simulink model "combined_models_v16"  (R2021a)
settings: Solver=VariableStepAuto  StartTime=0.0  StopTime=30  RelTol=1e-3
values from neighbouring files (symbols this model uses):
  r__s_st = r__s_stCG - r__t_tCG    [init_saildrone_dynamics_v5.m]    (also in moduleBasedModel_v7.m = cfg.r__s_st; systemVelocities.m = cfg.r__s_st)
  r__t_tAC = r__t_tCG    [init_saildrone_dynamics_v5.m]
  rho = 1025    [init_saildrone_dynamics_v5.m]    (also in moduleBasedModel_v7.m = cfg.rho; simplifiedModel_v8.m = cfg.rho)
  rho_air = 1.225    [init_saildrone_dynamics_v5.m]
undefined symbols (not defined in the file or in its folder): beta_V_w, cfg, delta_LOS, DiscIntNeverNeededParam, gamma_c, GWP, heading_controller_samplingtime, heading_rate_ref, K_b, K_d_heading, K_d_heading2, K_d_s, k_d_s, K_d_t, K_i_heading, K_i_heading2, K_i_s, k_i_s, K_i_t, K_p_heading, K_p_heading2, k_p_s, K_p_s, K_p_t, Ka_lin, keel, ObjectsPosition, omega_n_heading2, omega_n_s, q0, q_dot0, rudder, sail, sail_AOA_controller_samplingtime, sail_AOA_linearization_point, sail_AOA_saturation, sail_AOA_table, simulation_sampling_time, start_w_trans, tacking_minus, tacking_plus, tail, theta0, timeconstant_w, U_c, U_linearization_heading, U_w, U_w_step, v_current, v_wind, v_wind_unit, wn_ref_heading, wn_ref_t, xi0, zeta_ref_heading, zeta_ref_t
(part 2 of 3)

== system combined_models_v16/Subsystem/1st order rudder dynamics ==
  note: Create smooth saturation limits
  note: Positive rudder command
      | give positive heading angle
  note: Saturate angle input, so the derivative converge to 0 at saturation,
      | LP filter in order to maintain reasonable angular velocities
  delta_r0 : Inport
  delta_r_d : Inport  Port=2
  1/time constant : Gain  Gain=1/cfg.rudder_time_constant
  Integrator5 : Integrator  InitialConditionSource=external  InitialCondition=0.5
  Pos rudder give pos yaw : Gain  Gain=-1
  Saturation : Saturate  UpperLimit=cfg.rudder_saturation_limit  LowerLimit=-cfg.rudder_saturation_limit
  Saturation1 : Saturate  UpperLimit=cfg.rudder_saturation_limit  LowerLimit=-cfg.rudder_saturation_limit
  Sum6 : Sum  Inputs=|+-
  Transfer Fcn : TransferFcn  Denominator=[cfg.rudder_time_constant/10 1]
  Transfer Fcn1 : TransferFcn  Denominator=[cfg.rudder_time_constant/10 1]
  rudder gain : Gain  Gain=cfg.rudder_gain
  delta_r_dot : Outport
  delta_r : Outport  Port=2
  wires:
  Sum6/1 -> 1/time constant/1
  Integrator5/1 -> Saturation/1
  delta_r0/1 -> Integrator5/2
  delta_r_d/1 -> Pos rudder give pos yaw/1
  Saturation/1 -> Transfer Fcn/1
  Transfer Fcn/1 -> Sum6/2, delta_r/1
  Pos rudder give pos yaw/1 -> rudder gain/1
  1/time constant/1 -> delta_r_dot/1, Integrator5/1  "delta_r_dot"
  rudder gain/1 -> Saturation1/1
  Saturation1/1 -> Transfer Fcn1/1
  Transfer Fcn1/1 -> Sum6/1

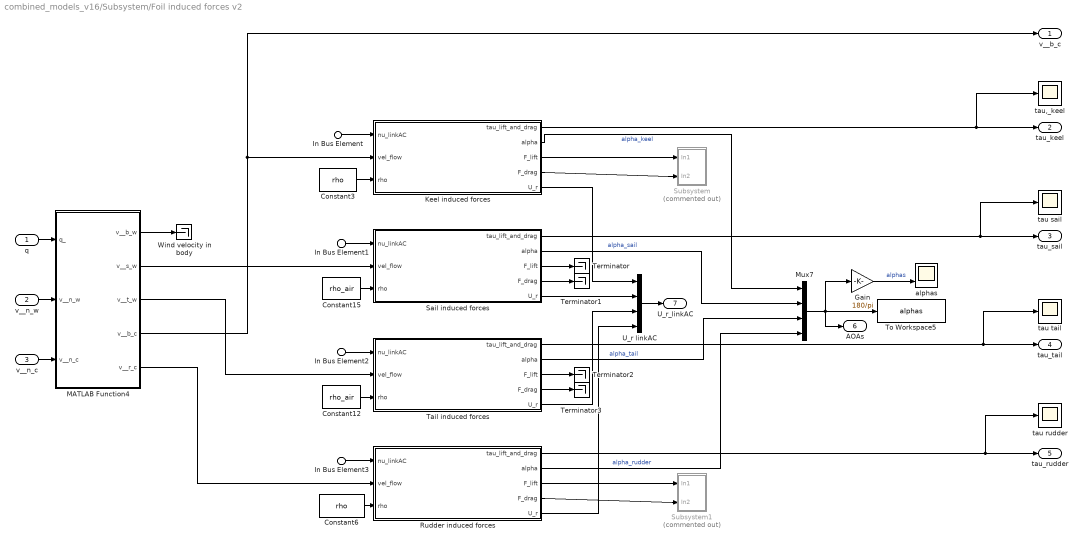
== system combined_models_v16/Subsystem/Foil induced forces v2 ==
  q : Inport
  v__n_w : Inport  Port=2
  v__n_c : Inport  Port=3
  In Bus Element : Inport  Port=4  PortName=nu_linkAC  Element=nu_keelAC
  In Bus Element1 : Inport  Port=4  PortName=nu_linkAC  Element=nu_sailAC
  In Bus Element2 : Inport  Port=4  PortName=nu_linkAC  Element=nu_tailAC
  In Bus Element3 : Inport  Port=4  PortName=nu_linkAC  Element=nu_rudderAC
  Constant12 : Constant  Value=rho_air
  Constant15 : Constant  Value=rho_air
  Constant3 : Constant  Value=rho
  Constant6 : Constant  Value=rho
  Gain : Gain  Gain=180/pi
  Keel induced forces : MATLAB Function  TreatAsAtomicUnit=on
  MATLAB Function4 : MATLAB Function  TreatAsAtomicUnit=on
  Mux7 : Mux
  Rudder induced forces : MATLAB Function  TreatAsAtomicUnit=on
  Sail induced forces : MATLAB Function  TreatAsAtomicUnit=on
  Subsystem : Subsystem  Commented=on
  Subsystem1 : Subsystem  Commented=on
  Tail induced forces : MATLAB Function  TreatAsAtomicUnit=on
  Terminator{,1..3} (4 alike) : Terminator
  To Workspace5 : ToWorkspace  VariableName=alphas  SampleTime=-1
  U_r linkAC : Mux
  Wind velocity in body : Terminator
  alphas : Scope  NumInputPorts=2
  tau rudder : Scope
  tau sail : Scope
  tau tail : Scope
  tau,_keel : Scope
  v__b_c : Outport
  tau_keel : Outport  Port=2
  tau_sail : Outport  Port=3
  tau_tail : Outport  Port=4
  tau_rudder : Outport  Port=5
  AOAs : Outport  Port=6
  U_r_linkAC : Outport  Port=7
  wires:
  Constant15/1 -> Sail induced forces/3(rho)
  Tail induced forces/1(tau_lift_and_drag) -> tau_tail/1, tau tail/1
  Mux7/1 -> AOAs/1, Gain/1, To Workspace5/1
  Sail induced forces/1(tau_lift_and_drag) -> tau_sail/1, tau sail/1
  MATLAB Function4/2(v__s_w) -> Sail induced forces/2(vel_flow)
  Constant12/1 -> Tail induced forces/3(rho)
  MATLAB Function4/3(v__t_w) -> Tail induced forces/2(vel_flow)
  In Bus Element2/1 -> Tail induced forces/1(nu_linkAC)
  Tail induced forces/2(alpha) -> Mux7/3  "alpha_tail"
  q/1 -> MATLAB Function4/1(q_)
  v__n_w/1 -> MATLAB Function4/2(v__n_w)
  In Bus Element1/1 -> Sail induced forces/1(nu_linkAC)
  v__n_c/1 -> MATLAB Function4/3(v__n_c)
  Sail induced forces/2(alpha) -> Mux7/2  "alpha_sail"
  In Bus Element/1 -> Keel induced forces/1(nu_linkAC)
  Constant3/1 -> Keel induced forces/3(rho)
  MATLAB Function4/4(v__b_c) -> v__b_c/1, Keel induced forces/2(vel_flow)
  Keel induced forces/1(tau_lift_and_drag) -> tau_keel/1, tau,_keel/1
  Keel induced forces/2(alpha) -> Mux7/1  "alpha_keel"
  Constant6/1 -> Rudder induced forces/3(rho)
  In Bus Element3/1 -> Rudder induced forces/1(nu_linkAC)
  MATLAB Function4/5(v__r_c) -> Rudder induced forces/2(vel_flow)
  Rudder induced forces/2(alpha) -> Mux7/4  "alpha_rudder"
  MATLAB Function4/1(v__b_w) -> Wind velocity in body/1
  Rudder induced forces/1(tau_lift_and_drag) -> tau_rudder/1, tau rudder/1
  Gain/1 -> alphas/2  "alphas"
  Keel induced forces/5(U_r) -> U_r linkAC/1
  Sail induced forces/5(U_r) -> U_r linkAC/2
  Tail induced forces/5(U_r) -> U_r linkAC/3
  Rudder induced forces/5(U_r) -> U_r linkAC/4
  Sail induced forces/3(F_lift) -> Terminator/1
  Sail induced forces/4(F_drag) -> Terminator1/1
  Tail induced forces/3(F_lift) -> Terminator2/1
  Tail induced forces/4(F_drag) -> Terminator3/1
  Keel induced forces/3(F_lift) -> Subsystem/1(In1)
  Keel induced forces/4(F_drag) -> Subsystem/2(In2)
  Rudder induced forces/3(F_lift) -> Subsystem1/1(In1)
  Rudder induced forces/4(F_drag) -> Subsystem1/2(In2)
  U_r linkAC/1 -> U_r_linkAC/1

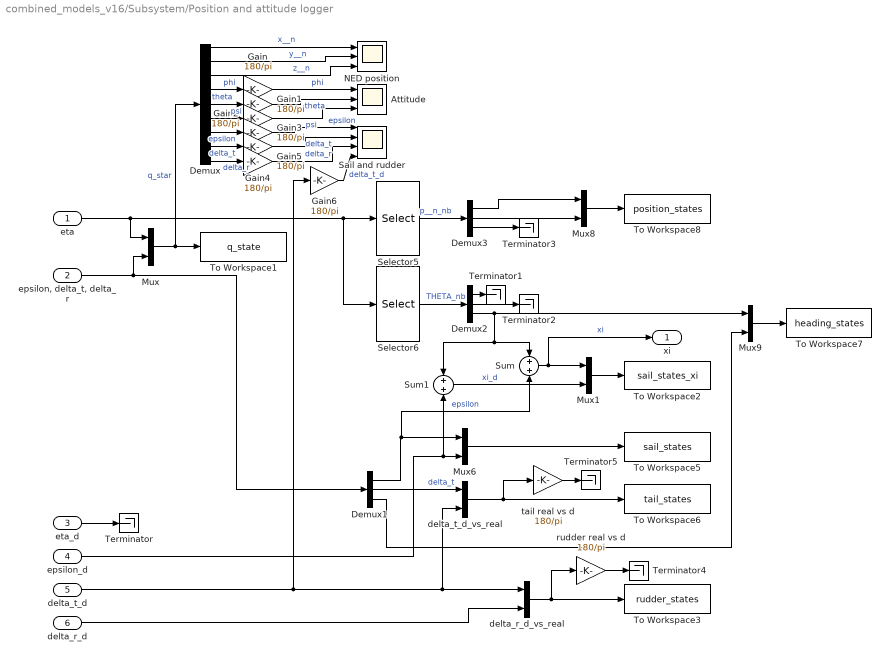
== system combined_models_v16/Subsystem/Position and attitude logger ==
  eta : Inport
  "epsilon, delta_t, delta_r" : Inport  Port=2
  eta_d : Inport  Port=3
  epsilon_d : Inport  Port=4
  delta_t_d : Inport  Port=5
  delta_r_d : Inport  Port=6
  Attitude : Scope  NumInputPorts=3
  Demux : Demux  Outputs=9
  Demux1 : Demux  Outputs=3
  Demux2 : Demux  Outputs=3
  Demux3 : Demux  Outputs=3
  Gain{,1..6} (7 alike) : Gain  Gain=180/pi
  Mux{,1,6,8..9} (5 alike) : Mux  Inputs=2
  NED position : Scope  NumInputPorts=3
  Sail and rudder : Scope  NumInputPorts=4
  Selector5 : Selector  InputPortWidth=6  IndexOptions=Index vector (dialog)  Indices=[1 2 3]  OutputSizes=1
  Selector6 : Selector  InputPortWidth=6  IndexOptions=Index vector (dialog)  Indices=[4 5 6]  OutputSizes=1
  Sum : Sum  Inputs=+|+
  Sum1 : Sum  Inputs=+|+
  Terminator{,1..5} (6 alike) : Terminator
  To Workspace1 : ToWorkspace  VariableName=q_state  SampleTime=-1
  To Workspace2 : ToWorkspace  VariableName=sail_states_xi  SampleTime=simulation_sampling_time
  To Workspace3 : ToWorkspace  VariableName=rudder_states  SampleTime=simulation_sampling_time
  To Workspace5 : ToWorkspace  VariableName=sail_states  SampleTime=simulation_sampling_time
  To Workspace6 : ToWorkspace  VariableName=tail_states  SampleTime=simulation_sampling_time
  To Workspace7 : ToWorkspace  VariableName=heading_states  SampleTime=simulation_sampling_time
  To Workspace8 : ToWorkspace  VariableName=position_states  SampleTime=simulation_sampling_time
  delta_r_d_vs_real : Mux  Inputs=2
  delta_t_d_vs_real : Mux  Inputs=2
  rudder real vs d : Gain  Gain=180/pi
  tail real vs d : Gain  Gain=180/pi
  xi : Outport
  wires:
  Demux2/3 -> Sum1/1, Sum/1, Mux9/1
  eta/1 -> Mux/1, Selector6/1, Selector5/1
  Demux3/1 -> Mux8/1
  Selector5/1 -> Demux3/1  "p__n_nb"
  Mux8/1 -> To Workspace8/1
  Mux9/1 -> To Workspace7/1
  Demux1/2 -> delta_t_d_vs_real/1  "delta_t"
  Demux3/2 -> Mux8/2
  Mux6/1 -> To Workspace5/1
  Selector6/1 -> Demux2/1  "THETA_nb"
  Demux1/1 -> Sum/2, Mux6/1  "epsilon"
  delta_t_d_vs_real/1 -> To Workspace6/1, tail real vs d/1
  "epsilon, delta_t, delta_r"/1 -> Mux/2, Demux1/1
  delta_t_d/1 -> Gain6/1, delta_t_d_vs_real/2, delta_r_d_vs_real/1
  epsilon_d/1 -> Mux6/2, Sum1/2
  eta_d/1 -> Terminator/1
  Demux2/2 -> Terminator2/1
  Demux2/1 -> Terminator1/1
  Demux3/3 -> Terminator3/1
  Mux/1 -> Demux/1, To Workspace1/1  "q_star"
  Gain4/1 -> Sail and rudder/2  "delta_t"
  Demux/2 -> NED position/2  "y__n"
  Demux/1 -> NED position/1  "x__n"
  Demux/3 -> NED position/3  "z__n"
  Gain3/1 -> Sail and rudder/1  "epsilon"
  Gain/1 -> Attitude/1  "phi"
  Gain1/1 -> Attitude/2  "theta"
  Gain2/1 -> Attitude/3  "psi"
  Demux1/3 -> Mux9/2
  Sum/1 -> xi/1, Mux1/1  "xi"
  Sum1/1 -> Mux1/2  "xi_d"
  Mux1/1 -> To Workspace2/1
  Demux/4 -> Gain/1  "phi"
  Demux/5 -> Gain1/1  "theta"
  Demux/6 -> Gain2/1  "psi"
  Demux/7 -> Gain3/1  "epsilon"
  Demux/8 -> Gain4/1  "delta_t"
  Demux/9 -> Gain5/1  "delta_r"
  Gain5/1 -> Sail and rudder/3  "delta_r"
  Gain6/1 -> Sail and rudder/4  "delta_t_d"
  delta_r_d/1 -> delta_r_d_vs_real/2
  tail real vs d/1 -> Terminator5/1
  delta_r_d_vs_real/1 -> rudder real vs d/1, To Workspace3/1
  rudder real vs d/1 -> Terminator4/1

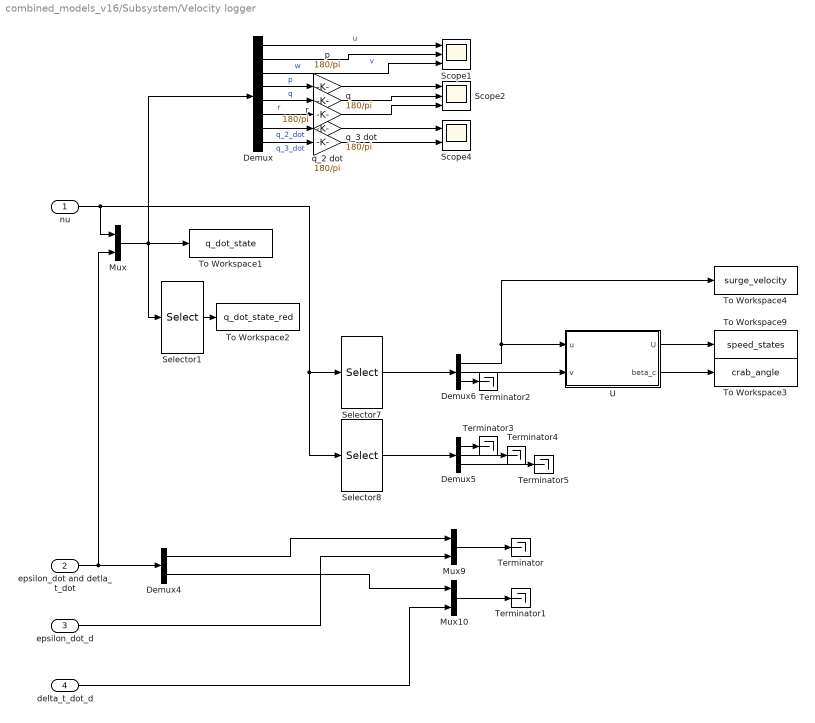
== system combined_models_v16/Subsystem/Velocity logger ==
  nu : Inport
  epsilon_dot and detla_t_dot : Inport  Port=2
  epsilon_dot_d : Inport  Port=3
  delta_t_dot_d : Inport  Port=4
  Demux : Demux  Outputs=8
  Demux4 : Demux  Outputs=2
  Demux5 : Demux  Outputs=3
  Demux6 : Demux  Outputs=3
  Mux : Mux  Inputs=2
  Mux10 : Mux  Inputs=2
  Mux9 : Mux  Inputs=2
  Scope1 : Scope  NumInputPorts=3
  Scope2 : Scope  NumInputPorts=3
  Scope4 : Scope  NumInputPorts=2
  Selector1 : Selector  InputPortWidth=8  IndexOptions=Index vector (dialog)  Indices=[1 2 4 6 7 8]  OutputSizes=1
  Selector7 : Selector  InputPortWidth=6  IndexOptions=Index vector (dialog)  Indices=[1 2 3]  OutputSizes=1
  Selector8 : Selector  InputPortWidth=6  IndexOptions=Index vector (dialog)  Indices=[4 5 6]  OutputSizes=1
  Terminator{,1..5} (6 alike) : Terminator
  To Workspace1 : ToWorkspace  VariableName=q_dot_state  SampleTime=-1
  To Workspace2 : ToWorkspace  VariableName=q_dot_state_red  SampleTime=simulation_sampling_time
  To Workspace3 : ToWorkspace  VariableName=crab_angle  SampleTime=simulation_sampling_time
  To Workspace4 : ToWorkspace  VariableName=surge_velocity  SaveFormat=Timeseries  SampleTime=simulation_sampling_time
  To Workspace9 : ToWorkspace  VariableName=speed_states  SampleTime=simulation_sampling_time
  U : MATLAB Function  TreatAsAtomicUnit=on
  p : Gain  Gain=180/pi
  q : Gain  Gain=180/pi
  q_2 dot : Gain  Gain=180/pi
  q_3 dot : Gain  Gain=180/pi
  r : Gain  Gain=180/pi
  wires:
  Selector8/1 -> Demux5/1
  Demux4/1 -> Mux9/1
  nu/1 -> Selector8/1, Selector7/1, Mux/1
  delta_t_dot_d/1 -> Mux10/2
  Demux4/2 -> Mux10/1
  Selector7/1 -> Demux6/1
  epsilon_dot_d/1 -> Mux9/2
  epsilon_dot and detla_t_dot/1 -> Demux4/1, Mux/2
  Demux6/1 -> To Workspace4/1, U/1(u)
  Demux6/2 -> U/2(v)
  U/1(U) -> To Workspace9/1
  Mux/1 -> To Workspace1/1, Demux/1, Selector1/1
  Demux/1 -> Scope1/1  "u"
  Demux/4 -> p/1  "p"
  Demux/5 -> q/1  "q"
  Demux/2 -> Scope1/2  "v"
  Demux/7 -> q_2 dot/1  "q_2_dot"
  Demux/3 -> Scope1/3  "w"
  Demux/8 -> q_3 dot/1  "q_3_dot"
  Demux/6 -> r/1  "r"
  Selector1/1 -> To Workspace2/1
  Mux9/1 -> Terminator/1
  Mux10/1 -> Terminator1/1
  Demux6/3 -> Terminator2/1
  Demux5/1 -> Terminator3/1
  Demux5/2 -> Terminator4/1
  Demux5/3 -> Terminator5/1
  U/2(beta_c) -> To Workspace3/1
  p/1 -> Scope2/1
  q/1 -> Scope2/2
  r/1 -> Scope2/3
  q_2 dot/1 -> Scope4/1
  q_3 dot/1 -> Scope4/2

== system combined_models_v16/Subsystem/v_wind ==
  Constant9 : Constant  Value=v_wind_unit
  MATLAB Function1 : MATLAB Function  TreatAsAtomicUnit=on
  Step : Step  Time=start_w_trans  Before=U_w  After=U_w+U_w_step  SampleTime=0
  Transfer Fcn : TransferFcn  Denominator=[timeconstant_w 1]
  y : Outport
  wires:
  Transfer Fcn/1 -> MATLAB Function1/1(a)
  Constant9/1 -> MATLAB Function1/2(b)
  MATLAB Function1/1(y) -> y/1
  Step/1 -> Transfer Fcn/1

== system combined_models_v16/Subsystem1/U_w ==
  Transfer Fcn1 : TransferFcn  Denominator=[timeconstant_w 1]
  U_w : Step  Time=start_w_trans  Before=U_w  After=U_w+U_w_step  SampleTime=0
  Out1 : Outport
  wires:
  U_w/1 -> Transfer Fcn1/1
  Transfer Fcn1/1 -> Out1/1

== system combined_models_v16/sail AOA control system/Gain scheduler1 ==
  note: discrete low
      | level controller
  AC relative velocity : Inport
  Constant1 : Constant  Value=K_b
  Constant2 : Constant  Value=k_p_s
  Constant3 : Constant  Value=omega_n_s
  MATLAB Function : MATLAB Function  TreatAsAtomicUnit=on
  Rate Transition5 : RateTransition  OutPortSampleTime=sail_AOA_controller_samplingtime
  Selector2 : Selector  InputPortWidth=4  IndexOptions=Index vector (dialog)  Indices=[2]  OutputSizes=1
  Transfer Fcn : TransferFcn  Denominator=[1 1]
  wn_ref_sAOA : Outport
  zeta_ref_sAOA : Outport  Port=2
  wires:
  Constant2/1 -> MATLAB Function/4(Kp)
  Constant1/1 -> MATLAB Function/3(Kb)
  Selector2/1 -> Rate Transition5/1  "sail AC velocity"
  Transfer Fcn/1 -> MATLAB Function/1(U_rw_sail)
  Rate Transition5/1 -> Transfer Fcn/1
  MATLAB Function/2(zeta_ref_sAOA) -> zeta_ref_sAOA/1
  AC relative velocity/1 -> Selector2/1
  MATLAB Function/1(wn_ref_sAOA) -> wn_ref_sAOA/1
  Constant3/1 -> MATLAB Function/2(omega_n_s)

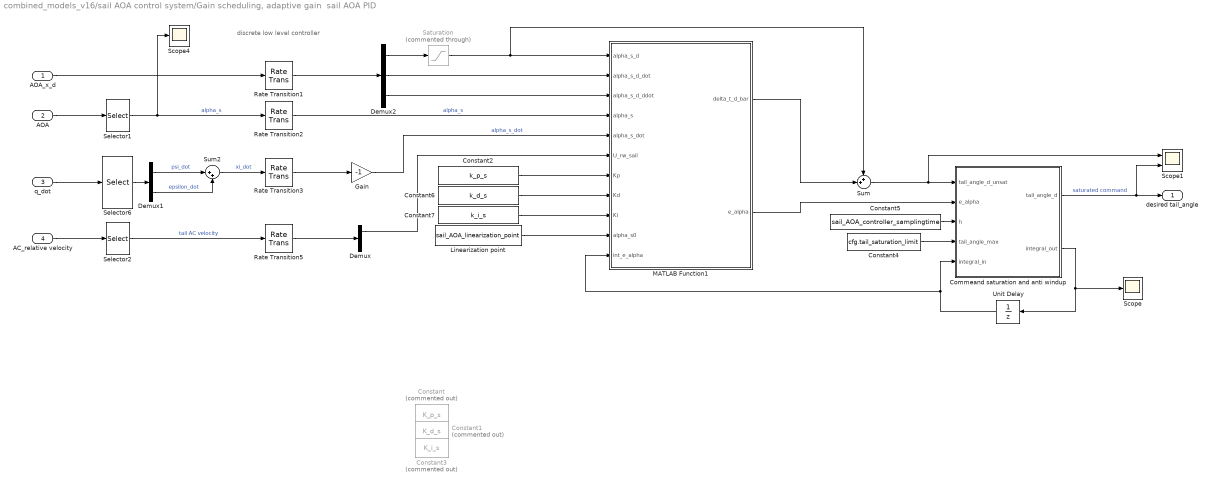
== system combined_models_v16/sail AOA control system/Gain scheduling, adaptive gain  sail AOA PID ==
  note: discrete low
      | level controller
  AOA_x_d : Inport
  AOA : Inport  Port=2
  q_dot : Inport  Port=3
  AC_relative velocity : Inport  Port=4
  Commeand saturation and anti windup : MATLAB Function  TreatAsAtomicUnit=on
  Constant : Constant  Commented=on  Value=K_p_s
  Constant1 : Constant  Commented=on  Value=K_d_s
  Constant2 : Constant  Value=k_p_s
  Constant3 : Constant  Commented=on  Value=K_i_s
  Constant4 : Constant  Value=cfg.tail_saturation_limit
  Constant5 : Constant  Value=sail_AOA_controller_samplingtime
  Constant6 : Constant  Value=k_d_s
  Constant7 : Constant  Value=k_i_s
  Demux : Demux  Outputs=2
  Demux1 : Demux  Outputs=2
  Demux2 : Demux  Outputs=3
  Gain : Gain  Gain=-1
  Linearization point : Constant  Value=sail_AOA_linearization_point
  MATLAB Function1 : MATLAB Function  TreatAsAtomicUnit=on
  Rate Transition{1..3,5} (4 alike) : RateTransition  OutPortSampleTime=sail_AOA_controller_samplingtime
  Saturation : Saturate  Commented=through  UpperLimit=sail_AOA_saturation  LowerLimit=-sail_AOA_saturation
  Scope : Scope
  Scope1 : Scope  NumInputPorts=2
  Scope4 : Scope
  Selector1 : Selector  InputPortWidth=4  IndexOptions=Index vector (dialog)  Indices=[2]  OutputSizes=1
  Selector2 : Selector  InputPortWidth=4  IndexOptions=Index vector (dialog)  Indices=[2 3]  OutputSizes=1
  Selector6 : Selector  InputPortWidth=8  IndexOptions=Index vector (dialog)  Indices=[6 7]  OutputSizes=1
  Sum : Sum  Inputs=++|
  Sum2 : Sum  Inputs=|++
  Unit Delay : UnitDelay  SampleTime=sail_AOA_controller_samplingtime  HasFrameUpgradeWarning=on
  desired tail_angle : Outport
  wires:
  AOA/1 -> Selector1/1
  q_dot/1 -> Selector6/1
  AOA_x_d/1 -> Rate Transition1/1
  AC_relative velocity/1 -> Selector2/1
  Selector1/1 -> Scope4/1, Rate Transition2/1  "alpha_s"
  Selector2/1 -> Rate Transition5/1  "tail AC velocity"
  Selector6/1 -> Demux1/1
  Demux1/1 -> Sum2/1  "psi_dot"
  Demux1/2 -> Sum2/2  "epsilon_dot"
  Sum2/1 -> Rate Transition3/1  "xi_dot"
  Rate Transition5/1 -> Demux/1
  Rate Transition3/1 -> Gain/1
  Gain/1 -> MATLAB Function1/5(alpha_s_dot)  "alpha_s_dot"
  Rate Transition1/1 -> Demux2/1
  Demux2/1 -> Saturation/1
  Demux2/2 -> MATLAB Function1/2(alpha_s_d_dot)
  Demux2/3 -> MATLAB Function1/3(alpha_s_d_ddot)
  Rate Transition2/1 -> MATLAB Function1/4(alpha_s)  "alpha_s"
  Demux/1 -> MATLAB Function1/6(U_rw_sail)
  Linearization point/1 -> MATLAB Function1/10(alpha_s0)
  MATLAB Function1/1(delta_t_d_bar) -> Sum/2
  MATLAB Function1/2(e_alpha) -> Commeand saturation and anti windup/2(e_alpha)
  Saturation/1 -> MATLAB Function1/1(alpha_s_d), Sum/1
  Constant6/1 -> MATLAB Function1/8(Kd)
  Constant2/1 -> MATLAB Function1/7(Kp)
  Constant7/1 -> MATLAB Function1/9(Ki)
  Sum/1 -> Scope1/1, Commeand saturation and anti windup/1(tail_angle_d_unsat)
  Constant4/1 -> Commeand saturation and anti windup/4(tail_angle_max)
  Constant5/1 -> Commeand saturation and anti windup/3(h)
  Unit Delay/1 -> MATLAB Function1/11(int_e_alpha), Commeand saturation and anti windup/5(integral_in)
  Commeand saturation and anti windup/2(integral_out) -> Scope/1, Unit Delay/1
  Commeand saturation and anti windup/1(tail_angle_d) -> Scope1/2, desired tail_angle/1  "saturated command"

== system combined_models_v16/sail AOA control system/Sail AOA reference model1 ==
  reference : Inport
  natraul_frequency : Inport  Port=2
  damping ratio : Inport  Port=3
  Constant2 : Constant  Value=[0;0;0]
  Demux : Demux  Outputs=3
  Integrator : Integrator  InitialConditionSource=external
  MATLAB Function : MATLAB Function  TreatAsAtomicUnit=on
  Terminator : Terminator
  Terminator1 : Terminator
  x_d : Outport
  ref : Outport  Port=2
  wires:
  MATLAB Function/1(x_refmod_dot) -> Integrator/1
  reference/1 -> MATLAB Function/1(reference)
  Integrator/1 -> x_d/1, MATLAB Function/4(x_refmod), Demux/1
  damping ratio/1 -> MATLAB Function/2(zeta_ref)
  natraul_frequency/1 -> MATLAB Function/3(wn_ref)
  Constant2/1 -> Integrator/2
  Demux/2 -> Terminator/1
  Demux/3 -> Terminator1/1
  Demux/1 -> ref/1

== system combined_models_v16/sailsystem dynamics2/1st order tail dynamics ==
  note: Create smooth saturation limits
  note: Saturate angle input, so the derivative converge to 0 at saturation,
      | LP filter in order to maintain reasonable angular velocities
  delta_t0 : Inport
  delta_t_d : Inport  Port=2
  1/time constant : Gain  Gain=1/cfg.tail_time_constant
  Integrator5 : Integrator  InitialConditionSource=external  InitialCondition=0.5
  Saturation : Saturate  UpperLimit=cfg.tail_saturation_limit  LowerLimit=-cfg.tail_saturation_limit
  Saturation1 : Saturate  UpperLimit=cfg.tail_saturation_limit  LowerLimit=-cfg.tail_saturation_limit  LinearizeAsGain=off
  Sum6 : Sum  Inputs=|+-
  Transfer Fcn : TransferFcn  Commented=through  Denominator=[cfg.tail_saturation_limit/10 1]
  Transfer Fcn1 : TransferFcn  Denominator=[cfg.tail_time_constant/10 1]
  tail gain : Gain  Gain=cfg.tail_gain
  delta_t_dot : Outport
  delta_t : Outport  Port=2
  wires:
  Sum6/1 -> 1/time constant/1
  Integrator5/1 -> Saturation/1
  delta_t0/1 -> Integrator5/2
  Saturation/1 -> Transfer Fcn/1
  Transfer Fcn/1 -> Sum6/2, delta_t/1
  delta_t_d/1 -> tail gain/1
  1/time constant/1 -> delta_t_dot/1, Integrator5/1  "delta_r_dot"
  tail gain/1 -> Saturation1/1
  Saturation1/1 -> Transfer Fcn1/1
  Transfer Fcn1/1 -> Sum6/1

== system combined_models_v16/sailsystem dynamics2/Sailsystem dynamics ==
  delta_t : Inport
  v__n_rw : Inport  Port=2
  Constant20 : Constant  Value=q_dot0(6)+q_dot0(7)
  Constant21 : Constant  Value=cfg.r__s_stAC
  Constant22 : Constant  Value=tail.K_C_L
  Constant23 : Constant  Value=cfg.I__PP_sailsystem(3,3)
  Demux : Demux  Outputs=2
  Integrator7 : Integrator  InitialConditionSource=external
  MATLAB Function5 : MATLAB Function  TreatAsAtomicUnit=on
  Mux10 : Mux  Inputs=2
  xi = psi + epsilon : Constant  Value=xi0
  beta_U_rw : Outport
  xi : Outport  Port=2
  xi_dot : Outport  Port=3
  wires:
  MATLAB Function5/2(beta_U_rw) -> beta_U_rw/1  "beta_U_rw"
  MATLAB Function5/1(x_dot) -> Integrator7/1
  xi = psi + epsilon/1 -> Mux10/1
  Integrator7/1 -> MATLAB Function5/1(x), Demux/1
  v__n_rw/1 -> MATLAB Function5/2(v__n_rw)
  Constant20/1 -> Mux10/2
  Constant21/1 -> MATLAB Function5/4(r__s_stAC)
  Mux10/1 -> Integrator7/2
  Constant22/1 -> MATLAB Function5/5(K_CL)
  Constant23/1 -> MATLAB Function5/6(I_zz_ss)
  Demux/1 -> xi/1  "xi"
  delta_t/1 -> MATLAB Function5/3(delta_t)
  Demux/2 -> xi_dot/1  "xi_dot"

== system combined_models_v16/sailsystem dynamics2/Subsystem ==
  beta_U_r : Inport
  xi_lin : Inport  Port=2
  v__n_rw : Inport  Port=3
  Constant22 : Constant  Value=rho_air
  Demux : Demux  Outputs=6
  Divide : Product  Inputs=*/
  Gain : Gain  Gain=180/pi
  MATLAB Function4 : MATLAB Function  TreatAsAtomicUnit=on
  alpha sail lin : Scope
  lift/drag in sail : Scope
  tau sail lin : Scope
  tau_sailsystem : Outport
  wires:
  Constant22/1 -> MATLAB Function4/4(rho_air)
  xi_lin/1 -> MATLAB Function4/2(xi)
  v__n_rw/1 -> MATLAB Function4/3(v__n_rw)
  beta_U_r/1 -> MATLAB Function4/1(beta_U_r)
  Demux/1 -> Divide/2
  Demux/2 -> Divide/1
  Divide/1 -> lift/drag in sail/1
  MATLAB Function4/1(tau_sailsystem) -> tau sail lin/1, tau_sailsystem/1, Demux/1
  MATLAB Function4/2(alpha_sail) -> Gain/1
  Gain/1 -> alpha sail lin/1

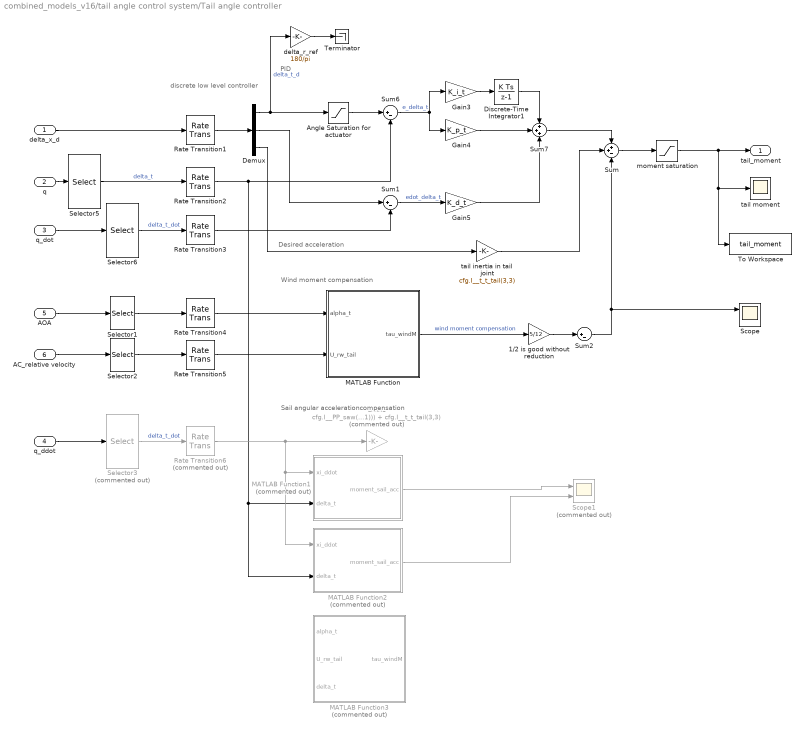
== system combined_models_v16/tail angle control system/Tail angle controller ==
  note: Desired acceleration
  note: Wind moment compensation
  note: PID
  note: discrete low
      | level controller
  note: Sail angular accelerationcompensation
  delta_x_d : Inport
  q : Inport  Port=2
  q_dot : Inport  Port=3
  q_ddot : Inport  Port=4
  AOA : Inport  Port=5
  AC_relative velocity : Inport  Port=6
  1/2 is good without reduction : Gain  Gain=5/12
  Angle Saturation for actuator : Saturate  UpperLimit=cfg.tail_saturation_limit  LowerLimit=-cfg.tail_saturation_limit
  Demux : Demux  Outputs=3
  Discrete-Time Integrator1 : DiscreteIntegrator  SampleTime=-1  ICPrevOutput=DiscIntNeverNeededParam  ICPrevScaledInput=DiscIntNeverNeededParam
  Gain1 : Gain  Commented=on  Gain=cfg.I__PP_saw(3,3)*(abs(r__t_tAC(1))/abs(r__s_st(1))) + cfg.I__t_t_tail(3,3)
  Gain3 : Gain  Gain=K_i_t
  Gain4 : Gain  Gain=K_p_t
  Gain5 : Gain  Gain=K_d_t
  MATLAB Function : MATLAB Function  TreatAsAtomicUnit=on
  MATLAB Function1 : MATLAB Function  Commented=on  TreatAsAtomicUnit=on
  MATLAB Function2 : MATLAB Function  Commented=on  TreatAsAtomicUnit=on
  MATLAB Function3 : MATLAB Function  Commented=on  TreatAsAtomicUnit=on
  Rate Transition{1..5} (5 alike) : RateTransition  OutPortSampleTime=lowel_moment_controller_samplingtime
  Rate Transition6 : RateTransition  Commented=on  OutPortSampleTime=lowel_moment_controller_samplingtime
  Scope : Scope  NumInputPorts=2
  Scope1 : Scope  Commented=on  NumInputPorts=2
  Selector1 : Selector  InputPortWidth=4  IndexOptions=Index vector (dialog)  Indices=[3]  OutputSizes=1
  Selector2 : Selector  InputPortWidth=4  IndexOptions=Index vector (dialog)  Indices=[2]  OutputSizes=1
  Selector3 : Selector  Commented=on  InputPortWidth=8  IndexOptions=Index vector (dialog)  Indices=[7]  OutputSizes=1
  Selector5 : Selector  InputPortWidth=9  IndexOptions=Index vector (dialog)  Indices=[8]  OutputSizes=1
  Selector6 : Selector  InputPortWidth=8  IndexOptions=Index vector (dialog)  Indices=[8]  OutputSizes=1
  Sum : Sum  Inputs=++-
  Sum1 : Sum  Inputs=|+-
  Sum2 : Sum  Inputs=|+-
  Sum6 : Sum  Inputs=|+-
  Sum7 : Sum  Inputs=+++
  Terminator : Terminator
  To Workspace : ToWorkspace  VariableName=tail_moment  SaveFormat=Timeseries  SampleTime=-1
  delta_r_ref : Gain  Gain=180/pi
  moment saturation : Saturate  UpperLimit=cfg.tail_moment_limit  LowerLimit=-cfg.tail_moment_limit
  tail inertia in tail joint : Gain  Gain=cfg.I__t_t_tail(3,3)
  tail moment : Scope
  tail_moment : Outport
  wires:
  Gain4/1 -> Sum7/2
  Rate Transition3/1 -> Sum1/2
  Sum6/1 -> Gain4/1, Gain3/1  "e_delta_t"
  Sum7/1 -> Sum/1
  Rate Transition2/1 -> MATLAB Function2/2(delta_t), MATLAB Function1/2(delta_t), Sum6/2
  Gain5/1 -> Sum7/3
  Rate Transition1/1 -> Demux/1
  Gain3/1 -> Discrete-Time Integrator1/1
  Discrete-Time Integrator1/1 -> Sum7/1
  q/1 -> Selector5/1
  q_dot/1 -> Selector6/1
  delta_x_d/1 -> Rate Transition1/1
  moment saturation/1 -> tail moment/1, To Workspace/1, tail_moment/1
  Angle Saturation for actuator/1 -> Sum6/1
  Demux/1 -> delta_r_ref/1, Angle Saturation for actuator/1  "delta_t_d"
  Sum1/1 -> Gain5/1  "edot_delta_t"
  AOA/1 -> Selector1/1
  AC_relative velocity/1 -> Selector2/1
  Rate Transition4/1 -> MATLAB Function/1(alpha_t)
  Sum/1 -> moment saturation/1
  Demux/2 -> Sum1/1
  Selector5/1 -> Rate Transition2/1  "delta_t"
  Selector6/1 -> Rate Transition3/1  "delta_t_dot"
  Demux/3 -> tail inertia in tail joint/1
  Selector1/1 -> Rate Transition4/1
  Selector2/1 -> Rate Transition5/1
  tail inertia in tail joint/1 -> Sum/2
  q_ddot/1 -> Selector3/1
  Selector3/1 -> Rate Transition6/1  "delta_t_dot"
  MATLAB Function/1(tau_windM) -> 1/2 is good without reduction/1  "wind moment compensation"
  Rate Transition6/1 -> Gain1/1, MATLAB Function2/1(xi_ddot), MATLAB Function1/1(xi_ddot)
  MATLAB Function1/1(moment_sail_acc) -> Scope1/1
  MATLAB Function2/1(moment_sail_acc) -> Scope1/2
  Sum2/1 -> Sum/3, Scope/1
  1/2 is good without reduction/1 -> Sum2/1
  Rate Transition5/1 -> MATLAB Function/2(U_rw_tail)
  delta_r_ref/1 -> Terminator/1

== system combined_models_v16/tail angle control system/Tail angle reference model ==
  reference : Inport
  Constant : Constant  Value=wn_ref_t
  Constant1 : Constant  Value=zeta_ref_t
  Constant2 : Constant  Value=[0;0;0]
  Demux : Demux  Outputs=3
  Integrator : Integrator  InitialConditionSource=external
  MATLAB Function : MATLAB Function  TreatAsAtomicUnit=on
  Scope : Scope
  Scope1 : Scope
  Terminator : Terminator
  Terminator1 : Terminator
  x_d : Outport
  delta_t_d : Outport  Port=2
  wires:
  MATLAB Function/1(x_refmod_dot) -> Integrator/1
  reference/1 -> Scope1/1, MATLAB Function/1(reference)
  Integrator/1 -> Scope/1, x_d/1, MATLAB Function/4(x_refmod), Demux/1
  Constant1/1 -> MATLAB Function/2(zeta_ref)
  Constant/1 -> MATLAB Function/3(wn_ref)
  Constant2/1 -> Integrator/2
  Demux/2 -> Terminator/1
  Demux/3 -> Terminator1/1
  Demux/1 -> delta_t_d/1

== system combined_models_v16/Heading PD control system1/Subsystem/heading reference model ==
  reference : Inport
  Constant : Constant  Value=wn_ref_heading
  Constant1 : Constant  Value=zeta_ref_heading
  Constant2 : Constant  Value=[theta0;0;0]
  Demux : Demux  Outputs=3
  Integrator : Integrator  InitialConditionSource=external
  MATLAB Function : MATLAB Function  TreatAsAtomicUnit=on
  Scope : Scope
  Scope1 : Scope
  Scope2 : Scope  NumInputPorts=2
  Terminator : Terminator
  Terminator1 : Terminator
  rate saturated ref model : Subsystem
  x_d : Outport
  delta_r_d : Outport  Port=2
  wires:
  MATLAB Function/1(x_refmod_dot) -> Integrator/1
  reference/1 -> rate saturated ref model/1(ref), Scope1/1, MATLAB Function/1(reference)
  Integrator/1 -> x_d/1, Scope/1, Scope2/2, MATLAB Function/4(x_refmod), Demux/1
  Constant1/1 -> MATLAB Function/2(zeta_ref)
  Constant/1 -> MATLAB Function/3(wn_ref)
  Constant2/1 -> Integrator/2
  Demux/2 -> Terminator/1
  Demux/3 -> Terminator1/1
  Demux/1 -> delta_r_d/1
  rate saturated ref model/1(desired) -> Scope2/1

== system combined_models_v16/Heading PD control system1/heading reference model1/rate saturated ref model ==
  ref : Inport
  Gain : Gain  Gain=wn_ref_heading
  Gain1 : Gain  Gain=wn_ref_heading^2
  Gain2 : Gain  Gain=wn_ref_heading^2
  Gain3 : Gain  Gain=2*zeta_ref_heading*wn_ref_heading
  Integrator1 : Integrator
  Integrator2 : Integrator
  Integrator3 : Integrator
  Mux : Mux  Inputs=3
  Saturation : Saturate  UpperLimit=heading_rate_ref  LowerLimit=-heading_rate_ref
  Sum : Sum  Inputs=|+-
  Sum1 : Sum  Inputs=|+-
  Sum2 : Sum  Inputs=|+-
  desired : Outport
  wires:
  Integrator1/1 -> Gain1/1, Sum/2
  Gain2/1 -> Sum1/2
  Integrator2/1 -> Mux/2, Gain3/1, Saturation/1
  Sum2/1 -> Mux/3, Integrator2/1
  Sum1/1 -> Sum2/1
  Gain/1 -> Integrator1/1
  Integrator3/1 -> Mux/1, Gain2/1
  Saturation/1 -> Integrator3/1
  Mux/1 -> desired/1
  Gain1/1 -> Sum1/1
  Sum/1 -> Gain/1
  Gain3/1 -> Sum2/2
  ref/1 -> Sum/1

== system combined_models_v16/Subsystem/Foil induced forces v2/Subsystem ==
  In1 : Inport
  In2 : Inport  Port=2
  Divide2 : Product  Commented=on  Inputs=*/
  lift/drag keel : Scope  Commented=on
  tau in flow keel : Scope  Commented=on  NumInputPorts=2
  wires:
  In2/1 -> tau in flow keel/1, Divide2/2
  Divide2/1 -> lift/drag keel/1
  In1/1 -> tau in flow keel/2, Divide2/1

== system combined_models_v16/Subsystem/Foil induced forces v2/Subsystem1 ==
  In1 : Inport
  In2 : Inport  Port=2
  Divide3 : Product  Commented=on  Inputs=*/
  lift/drag rudder : Scope  Commented=on
  tau in flow rudder : Scope  Commented=on  NumInputPorts=2
  wires:
  In2/1 -> Divide3/2, tau in flow rudder/1
  Divide3/1 -> lift/drag rudder/1
  In1/1 -> tau in flow rudder/2, Divide3/1

== system combined_models_v16/Heading PD control system1/Subsystem/heading reference model/rate saturated ref model ==
  ref : Inport
  Gain : Gain  Gain=wn_ref_heading
  Gain1 : Gain  Gain=wn_ref_heading^2
  Gain2 : Gain  Gain=wn_ref_heading^2
  Gain3 : Gain  Gain=2*zeta_ref_heading*wn_ref_heading
  Integrator1 : Integrator
  Integrator2 : Integrator
  Integrator3 : Integrator
  Mux : Mux  Inputs=3
  Saturation : Saturate  UpperLimit=heading_rate_ref  LowerLimit=-heading_rate_ref
  Sum : Sum  Inputs=|+-
  Sum1 : Sum  Inputs=|+-
  Sum2 : Sum  Inputs=|+-
  desired : Outport
  wires:
  Integrator1/1 -> Gain1/1, Sum/2
  Gain2/1 -> Sum1/2
  Integrator2/1 -> Mux/2, Gain3/1, Saturation/1
  Sum2/1 -> Mux/3, Integrator2/1
  Sum1/1 -> Sum2/1
  Gain/1 -> Integrator1/1
  Integrator3/1 -> Mux/1, Gain2/1
  Saturation/1 -> Integrator3/1
  Mux/1 -> desired/1
  Gain1/1 -> Sum1/1
  Sum/1 -> Gain/1
  Gain3/1 -> Sum2/2
  ref/1 -> Sum/1

== matlab function combined_models_v16/tail angle control system/Tail angle controller/MATLAB Function1 ==
  data: xi_ddot input; moment_sail_acc output; delta_t input; cfg parameter
function moment_sail_acc = fcn(xi_ddot, delta_t, cfg)

    moment_sail_acc = xi_ddot*(cfg.I__PP_saw(3,3)*(abs(cfg.r__t_tAC(1))/(abs(cfg.r__s_st(1))*cos(delta_t))) + cfg.I__t_t_tail(3,3));

== matlab function combined_models_v16/tail angle control system/Tail angle controller/MATLAB Function2 ==
  data: xi_ddot input; moment_sail_acc output; delta_t input; cfg parameter
function moment_sail_acc = fcn(xi_ddot, delta_t, cfg)

%     moment_sail_acc = xi_ddot*(cfg.I__PP_saw(3,3)*cfg.I__t_t_tail(3,3))/(cfg.m_tail*(abs(cfg.r__s_st(1))^2));
%     moment_sail_acc = xi_ddot*0.43;

% moment_sail_acc = xi_ddot*((   cfg.I__PP_saw(3,3) + cfg.I__t_t_tail(3,3) + cfg.m_tail*abs(cfg.r__s_st(1))^2)*cfg.I__t_t_tail(3,3))/(cfg.m_tail*(abs(cfg.r__s_st(1))^2));
moment_sail_acc = xi_ddot*(cfg.I__PP_sailsystem(3,3)*cfg.I__t_t_tail(3,3))/(cfg.m_tail*(abs(cfg.r__s_st(1))^2))

== matlab function combined_models_v16/tail angle control system/Tail angle controller/MATLAB Function3 ==
  data: alpha_t input; U_rw_tail input; delta_t input; tau_windM output; cfg parameter; tail parameter
function tau_windM = windMoment(alpha_t,U_rw_tail, delta_t, cfg, tail)

% Distance from actuator axis to AC of tail:
l_s_st = abs(cfg.r__s_st(1));

tau_windM = tail.K_C_L*(U_rw_tail^2)*sin(alpha_t)*l_s_st*cos(delta_t);

== matlab function combined_models_v16/Optimal sail AOA selector/MATLAB Function1 ==
  data: Cy input; alpha_k_d output; U_rw input; U_rc input; cfg parameter; keel parameter; sail parameter
function alpha_k_d = sideSlipController(Cy,U_rw, U_rc, cfg, keel, sail)

% assuming relative velocity is mainly along ship, then a force in postive
% sway direction need to be compansated with a positive keel AOA (AOA defined with respect to keel/hull)

if U_rc>0.1
    alpha_k_d = ((U_rw^2)*cfg.rho_air*sail.S*Cy)/((U_rc^2)*cfg.rho*keel.S*keel.C_L_alpha);
else
    alpha_k_d = 0;
end

== matlab function combined_models_v16/Optimal sail AOA selector/MATLAB Function4 ==
  data: index input; modedindex output; last_index input; last_index output
function [modedindex, last_index] = alteringPrevention(index, last_index)

    threshold = 4;% 
    
    if last_index == -999
        % these are list spesific indexes taken from the sail_AOA_table
        if index == 58 
            last_index = 58;
            modedindex = index;
        elseif index == 61
            last_index = 61;
            modedindex = index;
        elseif index == 301
            last_index = 301;
            modedindex = index;
        elseif index == 304
            last_index = 304;
            modedindex = index;
        else
            modedindex = index;
        end
    else
        if (index > last_index + threshold)
            last_index = -999;
            modedindex = index;
        elseif (index < last_index - threshold)
            last_index = -999;
            modedindex = index;
        else
            modedindex = last_index;
        end
    end 
            
%     elseif ( && (last_index ~= -999)) % these will case bug when -99 hence protected by default case over
%         last_index = -999;
%         modedindex = index;
%     elseif ((index < last_index - threshold) && (last_index ~= -999))
%         last_index = -999;
%         modedindex = index;
%     elseif index == 58 % these are protected by the ifs over..........
%         last_index = 58;
%         modedindex = index;
%     elseif index == 61
%         last_index = 61;
%         modedindex = index;
%     else
%         error_flag = 1;
%     end


%     if ((index == 58) && (last_index == -999)) % these are protected by the ifs over..........
%         last_index = 58;
%         modedindex = index;
%     elseif index == 61
%         last_index = 61;
%         modedindex = index;    
% 
% 
%     if last_index == -999
%         modedindex = index;
%     elseif ((index > last_index + threshold) && (last_index ~= -999)) % these will case bug when -99 hence protected by default case over
%         last_index = -999;
%         modedindex = index;
%     elseif ((index < last_index - threshold) && (last_index ~= -999))
%         last_index = -999;
%         modedindex = index;
%     elseif index == 58 % these are protected by the ifs over..........
%         last_index = 58;
%         modedindex = index;
%     elseif index == 61
%         last_index = 61;
%         modedindex = index;
%     else
%         error_flag = 1;
%     end

== matlab function combined_models_v16/sail AOA control system/Sail AOA reference model1/MATLAB Function ==
  data: reference input; x_refmod_dot output; zeta_ref input; wn_ref input; x_refmod input
function x_refmod_dot  = refModelSailAOA(reference, zeta_ref, wn_ref, x_refmod)

[x_refmod_dot] = referenceModelPA(reference, zeta_ref, wn_ref, x_refmod);

== matlab function combined_models_v16/sail AOA control system/Gain scheduling, adaptive gain  sail AOA PID/Commeand saturation and anti windup ==
  data: tail_angle_d_unsat input; e_alpha input; h input; tail_angle_max input; tail_angle_d output; integral_in input; integral_out output
function [tail_angle_d, integral_out] = SatAndAntiWindUP(tail_angle_d_unsat, e_alpha, h, tail_angle_max, integral_in)


% function [tail_angle_d, integral_out] = SatAndAntiWindUP(tail_angle_d_unsat, e_alpha, U_rw_tail_star, U_rw_tail_star_prev, K_i_s, Kb, h, tail_angle_max, integral_in, cfg)
    % h = sampling time
    
    % is tail angle saturated?
    if abs(tail_angle_d_unsat)> tail_angle_max
        tail_angle_d = sign(tail_angle_d_unsat)*tail_angle_max;
        
        % if tail angle is saturated, simply stop integrating
        integral_out = integral_in;

    else
        tail_angle_d = tail_angle_d_unsat;
        % euler integration
        integral_out = integral_in + h*e_alpha;
    end

%     % euler integration
%     if sat_flag == 0
%         integral_out = integral_in + h*e_alpha;
%     else
%         % if tail angle is 
%         integral_out = integral_in;
%     end
    
    
    
        % cfg.I__PP_sailsystem due to way controller is defined (delta_t_d
        % = alpha_s_d + 1/K2(.......)) where delta_t_d is devided by cfg.I__PP_sailsystem(3,3)
%         integral = integral_in + (h*cfg.I__PP_sailsystem(3,3)/((U_rw_tail_star^3)*0.5*Kb*K_i_s))*(tail_angle_d-tail_angle_d_unsat);
%         integral = integral_in - (h/((U_rw_tail_star)*K_i_s))*(tail_angle_d-tail_angle_d_unsat);
%         integral = (U_rw_tail_star*integral_in - (h/((U_rw_tail_star)*K_i_s))*(tail_angle_d-tail_angle_d_unsat))/U_rw_tail_star_prev;
%         integral = integral_in - (h*cfg.I__PP_sailsystem(3,3)/(K_i_s))*(tail_angle_d-tail_angle_d_unsat);

== matlab function combined_models_v16/sail AOA control system/Gain scheduler1/MATLAB Function ==
  data: U_rw_sail input; omega_n_s input; Kb input; Kp input; wn_ref_sAOA output; zeta_ref_sAOA output; cfg parameter
function [wn_ref_sAOA, zeta_ref_sAOA] = GS(U_rw_sail, omega_n_s, Kb, Kp, cfg)

% Change reference model with velocity to adjust reference model to the
% sailsystems changing bandwidth 

               
omega_n_s = U_rw_sail*omega_n_s;%sqrt((-Kb*(U_rw_sail^2)*(1+Kp))/cfg.I__PP_sailsystem(3,3));
%% Sail AOA reference model

% adjust reference model with respect to current system dynnamics, allow
% 10% margin for tracking controll
wn_ref_sAOA = omega_n_s*0.6;
zeta_ref_sAOA = 1;

== matlab function combined_models_v16/Optimal sail AOA selector/MATLAB Function ==
  data: angle input; index output
function index = mapAngle2Index(angle)

    nr_indexes = 360; % number -1
    angle = ssa(angle); % make sure angle is in -pi to pi domain
    
    k = angle/(2*pi) + 0.5; % transform to 0 to 1
    
    index = 1 + round(k*nr_indexes);
    
%     if index <= 0
%         index
%     elseif index > nr_indexes + 1
%         index
%     end

== matlab function combined_models_v16/Optimal sail AOA selector/MATLAB Function3 ==
  data: v__n_sailAC_rel input; beta__n_rw output
function beta__n_rw = vSailAC2betarw(v__n_sailAC_rel)
    % use realtive velocity of sail with respect to wind in NED to calulate the angle of the relative velocity 

    beta__n_rw = atan2(v__n_sailAC_rel(2),v__n_sailAC_rel(1));

== matlab function combined_models_v16/sail AOA control system/Gain scheduling, adaptive gain  sail AOA PID/MATLAB Function1 ==
  data: alpha_s_d input; delta_t_d_bar output; alpha_s_d_dot input; alpha_s_d_ddot input; alpha_s input; alpha_s_dot input; U_rw_sail input; Kp input; Kd input; Ki input; alpha_s0 input; int_e_alpha input; tail parameter; cfg parameter; e_alpha output
function [delta_t_d_bar, e_alpha] = GSPID(alpha_s_d, alpha_s_d_dot, alpha_s_d_ddot, alpha_s, alpha_s_dot, U_rw_sail, Kp, Kd, Ki,alpha_s0, int_e_alpha, tail, cfg)
% the GS PID part of the controller

% stop adpting parameters to avoid high values
% U_rw_tail_star = max(U_rw_tail, 2); %7;max(U_rw_tail, 2);%15;%max(U_rw_tail, 2);
U_rw_sail_star = max(U_rw_sail, 2); %7;max(U_rw_tail, 2);%15;%max(U_rw_tail, 2);

Ka = (cfg.r__s_stAC(1)^2)*((cos(alpha_s0))^2)*tail.K_C_L;
Kb = cfg.r__s_stAC(1)*cos(alpha_s0)*tail.K_C_L;


e_alpha = alpha_s-alpha_s_d;
e_alpha_dot = alpha_s_dot-alpha_s_d_dot; 

% The controller (without the alpha_s_d feed forward)
delta_t_d_bar = -Ka*alpha_s_d_dot/(Kb*U_rw_sail_star) - Kd*e_alpha_dot/U_rw_sail_star - Kp*e_alpha - alpha_s_d_ddot*cfg.I__PP_sailsystem(3,3)/(Kb*U_rw_sail_star^2)- U_rw_sail_star*Ki*int_e_alpha;
% delta_t_d_bar = (1/K2)*(-cfg.I__PP_sailsystem(3,3)*alpha_s_d_ddot - K1*alpha_s_d_dot + Kd_star*e_alpha_dot + Kp_star*e_alpha + Ki*int_e_alpha);
% delta_t_d_bar = (1/K2)*(-cfg.I__PP_sailsystem(3,3)*alpha_s_d_ddot - K1*alpha_s_d_dot + Kd_star*e_alpha_dot + Kp*e_alpha);

%% antiwindup how will it be????


% shut down controller for small velocities, makes it a pure feed forward,
% need faiding here?
if U_rw_sail < 0.1
    delta_t_d_bar = 0;
end

% implement a set of alternative gain and faiding between?
% integrator and anti windup

% Faiding out the controller might not work with integrator?

== matlab function combined_models_v16/Subsystem/Crab angel ==
  data: q input; chi output; q_dot input; beta_crab output
function [chi, beta_crab]  = crabAngle(q, q_dot)

psi = q(6);


u = q_dot(1);
v = q_dot(2);
beta_crab = atan2(v,u); 

chi = psi + beta_crab;

== matlab function combined_models_v16/Optimal sail AOA selector/MATLAB Function2 ==
  data: C_x input; C_y input; U_rw_sail input; fx output; fy output; sail parameter
function [fx, fy] = sailForceEstimate(C_x, C_y, U_rw_sail, sail)
    % notice that this function can be used both with respect to the body
    % axes and the course axes


fx = sail.K_C_L*(U_rw_sail^2)*C_x;
fy = sail.K_C_L*(U_rw_sail^2)*C_y;

% % Distance from actuator axis to AC of tail:
% l_t_AC = abs(cfg.r__t_tAC(1));
% 
% tau_windM = tail.K_C_L*(U_rw_tail^2)*sin(alpha_t)*l_t_AC;

== matlab function combined_models_v16/Subsystem/Foil induced forces v2/Tail induced forces ==
  data: nu_linkAC input; tau_lift_and_drag output; vel_flow input; rho input; alpha output; F_lift output; F_drag output; tail parameter; U_r output
function [tau_lift_and_drag, alpha, F_lift, F_drag, U_r] = modelBasedLiftDragForces(nu_linkAC, vel_flow, rho, tail)

% take foil_param as a struct from workspace
foil_param = tail;
[tau_lift_and_drag, alpha, F_lift, F_drag, U_r] = modelBasedLiftDragForces_wmoment(nu_linkAC, vel_flow, rho, foil_param);

== matlab function combined_models_v16/Subsystem/Foil induced forces v2/Sail induced forces ==
  data: nu_linkAC input; tau_lift_and_drag output; vel_flow input; rho input; alpha output; F_lift output; F_drag output; sail parameter; U_r output
function [tau_lift_and_drag, alpha, F_lift, F_drag, U_r] = modelBasedLiftDragForces(nu_linkAC, vel_flow, rho, sail)

% take foil_param as a struct from workspace
foil_param = sail;
[tau_lift_and_drag, alpha, F_lift, F_drag, U_r] = modelBasedLiftDragForces_wmoment(nu_linkAC, vel_flow, rho, foil_param);

== matlab function combined_models_v16/Subsystem/Foil induced forces v2/Keel induced forces ==
  data: nu_linkAC input; tau_lift_and_drag output; vel_flow input; rho input; alpha output; F_lift output; F_drag output; keel parameter; U_r output
function [tau_lift_and_drag, alpha, F_lift, F_drag, U_r] = modelBasedLiftDragForces(nu_linkAC, vel_flow, rho, keel)

% take foil_param as a struct from workspace
foil_param = keel;
[tau_lift_and_drag, alpha, F_lift, F_drag, U_r] = modelBasedLiftDragForces_wmoment(nu_linkAC, vel_flow, rho, foil_param);

== matlab function combined_models_v16/Subsystem/Foil induced forces v2/MATLAB Function4 ==
  data: q_ input; v__b_w output; v__n_w input; v__n_c input; v__s_w output; v__t_w output; v__b_c output; v__r_c output
function [v__b_w, v__s_w, v__t_w, v__b_c, v__r_c]= flowVelocities(q_, v__n_w, v__n_c)

[v__b_w, v__s_w, v__t_w, v__b_c, v__r_c]= flowVelocities(q_, v__n_w, v__n_c);

== matlab function combined_models_v16/Subsystem/Foil induced forces v2/Rudder induced forces ==
  data: nu_linkAC input; tau_lift_and_drag output; vel_flow input; rho input; alpha output; F_lift output; F_drag output; rudder parameter; U_r output
function [tau_lift_and_drag, alpha, F_lift, F_drag, U_r] = modelBasedLiftDragForces(nu_linkAC, vel_flow, rho, rudder)

% take foil_param as a struct from workspace
foil_param = rudder;
[tau_lift_and_drag, alpha, F_lift, F_drag, U_r] = modelBasedLiftDragForces_wmoment(nu_linkAC, vel_flow, rho, foil_param);

== matlab function combined_models_v16/Crab angle and sway force compensation  ==
  data: psi_compensation input; heading_reference output; desired_course input; beta_crab input; AC_relative input
function heading_reference = fcn(psi_compensation,desired_course, beta_crab, AC_relative)

U_rc = AC_relative(1);

% faid function
sigma = 0.5+(1/pi)*atan(100*U_rc-30);

if U_rc < 0.05
    psi_compensation = 0;
    beta_crab = 0;
end

heading_reference = desired_course + sigma*(psi_compensation-beta_crab);

== matlab function combined_models_v16/WP Manager/MATLAB Function1 ==
  data: local_path_complete output; next_wp output size=2; prev_wp output size=2; next_wp_index output; q input; prev_wp_index output; WP input; next_wp_index input; prev_wp_index input; firstWP input; firstWP output
function [local_path_complete, next_wp ,prev_wp, next_wp_index, prev_wp_index, firstWP] = WPManager(q,WP, next_wp_index, prev_wp_index, firstWP)
% Switch waypoint when close enough => error norm (circle of acceptance)

% next_wp = zeros(2,1);
% prev_wp = zeros(2,1);

% check for new list
if WP(:,1) ~=  firstWP
    firstWP = WP(:,1)
    % reset indexes
    next_wp_index = 2;
    prev_wp_index = 1;
end
    

local_path_complete = 0;

% check circle of acceptance
next_wp = WP(:,next_wp_index);
position_error = [q(1); q(2)] - next_wp;
error_norm = sqrt(position_error(1)^2 + position_error(2)^2);

if isnan(WP(1,next_wp_index+1)) % when last WP
    circ_accept = 20;
else
    circ_accept = 10;%5%13;
end
    
if error_norm <= circ_accept
    prev_wp_index = next_wp_index;                      % set new wayspoints
    next_wp_index = next_wp_index + 1;
end

% Ask for next path
if isnan(WP(1,next_wp_index)) 
    % send old WP until further
    next_wp = WP(:,2); % for testing
    prev_wp = WP(:,1); % for testing
%     next_wp = WP(:,next_wp_index-1);
%     prev_wp = WP(:,prev_wp_index-1);
    
    % reset indexes
    next_wp_index = 2;
    prev_wp_index = 1;
    
    % ask for new WP
    local_path_complete = 1;
    
else
    % update and send 
    next_wp = WP(:,next_wp_index);
    prev_wp = WP(:,prev_wp_index);
end

== matlab function combined_models_v16/LOS/MATLAB Function2 ==
  data: next_wp input; chi_d output; prev_wp input; delta input; q input
function chi_d  = LOSguidance(next_wp, prev_wp, delta, q)
%GUIDENCE Summary of this function goes here
%   Find desired course based on LOS guidence law

eta = q(1:6);

% Guidance parameters
% delta = 40;%50; %look ahead distance
K_p = 1/delta;

% path tangential angle
pi_p = atan2(next_wp(2)-prev_wp(2), next_wp(1)-prev_wp(1));

% rotation matrix
R__n_p = [cos(pi_p) -sin(pi_p);
          sin(pi_p) cos(pi_p)];
      
% error in p-frame
error_p = R__n_p'*([eta(1); eta(2)] - prev_wp);
% cross track error
y__p_e = error_p(2);

chi_d = pi_p - atan(K_p*y__p_e);
end

== matlab function combined_models_v16/MATLAB Function10 ==
  data: eta input; nu input; eta_dot output
function eta_dot = J_THETA(eta,nu)
    % eta_dot = J_THETA(eta)*nu 2.53 FOSSEN

    phi = eta(4);
    theta = eta(5);
    psi = eta(6);
    
    J = eulerang(phi, theta, psi);
    
    eta_dot = J*nu;

== matlab function combined_models_v16/simplified vessel model ==
  data: q_ input; q_ddot output; q_dot input; v__n_c input; tau_sail input; delta_r input; cfg parameter; rudder parameter; keel parameter
function q_ddot = simplifiedVesselModel(q_, q_dot, v__n_c, tau_sail, delta_r, cfg, rudder, keel)

q_ddot = simplifiedModel_v8(q_, q_dot, v__n_c, tau_sail, delta_r, cfg, rudder, keel);

== matlab function combined_models_v16/Heading PD control system1/Subsystem/MATLAB Function3 ==
  data: u input; U_linearization_heading input; y output; rudder parameter; cfg parameter
function y  = fcn(u,U_linearization_heading,rudder, cfg)

% y = u/(-rudder.K_C_L*(cfg.r__b_brAC(1))*U_linearization_heading);
y = u/(-rudder.K_C_L*(cfg.r__b_brAC(1))*U_linearization_heading^2);

% rudderk = rudder.K_C_L;
% r__b = cfg.r__b_brAC(1);
% U_linearization_heading = U_linearization_heading;


% rudderk, r__b, U_linearization_heading

== matlab function combined_models_v16/tail angle control system/Tail angle reference model/MATLAB Function ==
  data: reference input; x_refmod_dot output; zeta_ref input; wn_ref input; x_refmod input
function x_refmod_dot  = refModelTail(reference, zeta_ref, wn_ref, x_refmod)

[x_refmod_dot] = referenceModelPA(reference, zeta_ref, wn_ref, x_refmod);

== matlab function combined_models_v16/Heading PD control system1/Commeand saturation and anti windup ==
  data: rudder_angle_d_unsat input; e_alpha input; h input; rudder_angle_max input; rudder_stall input; rudder_angle_d output; integral_in input; integral_out output
function [rudder_angle_d, integral_out] = SatAndAntiWindUP(rudder_angle_d_unsat, e_alpha, h, rudder_angle_max, rudder_stall, integral_in)


% function [tail_angle_d, integral_out] = SatAndAntiWindUP(tail_angle_d_unsat, e_alpha, U_rw_tail_star, U_rw_tail_star_prev, K_i_s, Kb, h, tail_angle_max, integral_in, cfg)
    % h = sampling time
    
    % is tail angle saturated?
    if abs(rudder_angle_d_unsat)> rudder_angle_max
        rudder_angle_d = sign(rudder_angle_d_unsat)*rudder_angle_max;
        
        % if tail angle is saturated, simply stop integrating
        integral_out = integral_in;
    elseif abs(rudder_angle_d_unsat)> rudder_stall
        % ordinary output
        rudder_angle_d = rudder_angle_d_unsat;
        
        % stop integrator at stall
        integral_out = integral_in;

    else
        rudder_angle_d = rudder_angle_d_unsat;
        % euler integration
        integral_out = integral_in + h*e_alpha;
    end

%     % euler integration
%     if sat_flag == 0
%         integral_out = integral_in + h*e_alpha;
%     else
%         % if tail angle is 
%         integral_out = integral_in;
%     end
    
    
    
        % cfg.I__PP_sailsystem due to way controller is defined (delta_t_d
        % = alpha_s_d + 1/K2(.......)) where delta_t_d is devided by cfg.I__PP_sailsystem(3,3)
%         integral = integral_in + (h*cfg.I__PP_sailsystem(3,3)/((U_rw_tail_star^3)*0.5*Kb*K_i_s))*(tail_angle_d-tail_angle_d_unsat);
%         integral = integral_in - (h/((U_rw_tail_star)*K_i_s))*(tail_angle_d-tail_angle_d_unsat);
%         integral = (U_rw_tail_star*integral_in - (h/((U_rw_tail_star)*K_i_s))*(tail_angle_d-tail_angle_d_unsat))/U_rw_tail_star_prev;
%         integral = integral_in - (h*cfg.I__PP_sailsystem(3,3)/(K_i_s))*(tail_angle_d-tail_angle_d_unsat);
